simulink model "Docking"  (R2024b)
settings: Solver=VariableStepAuto  StartTime=0.0  StopTime=inf  RelTol=1e-3
values from neighbouring files (symbols this model uses):
  mu = 3.986e14    (= 398600000000000)    [DockSimParams.m]
undefined symbols (not defined in the file or in its folder): prox, sat
libraries: matrix_library x3
settings Model: Creator=Ameya  LastModifiedBy=Ameya
settings RTWCC: GPUComputeCapability=3.5

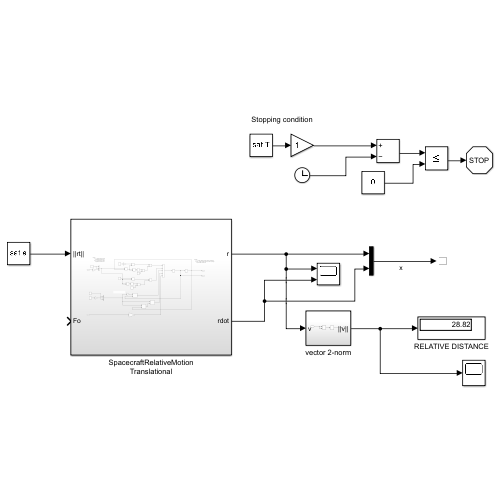
[thumbnail: Simulink's stored preview of the top-level diagram]
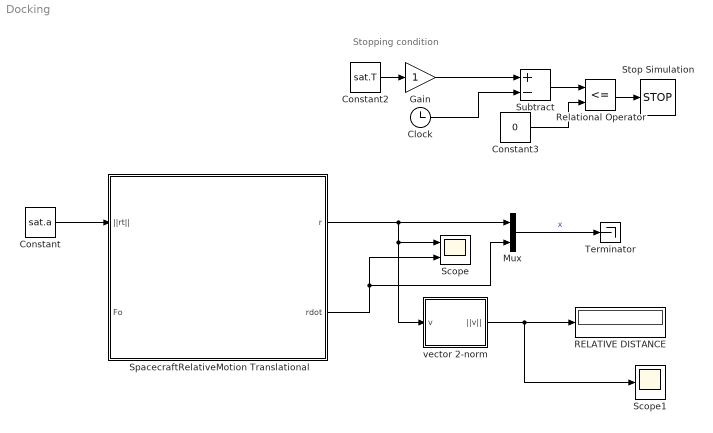
== system Docking ==
  note: Stopping condition
  Clock : Clock
  Constant : Constant  Value=sat.a
  Constant2 : Constant  Value=sat.T
  Constant3 : Constant  Value=0
  Gain : Gain
  Mux : Mux  Inputs=2
  RELATIVE DISTANCE : Display
  Relational Operator : RelationalOperator  Operator=<=  OutDataTypeStr=boolean  RndMeth=Simplest  InputSameDT=off
  Scope : Scope  NumInputPorts=2
  Scope1 : Scope
  SpacecraftRelativeMotion Translational : Subsystem
  Stop Simulation : Stop
  Subtract : Sum  Inputs=+-
  Terminator : Terminator
  vector 2-norm : Subsystem
  wires:
  SpacecraftRelativeMotion Translational/1(r) -> Mux/1, vector 2-norm/1(v), Scope/1
  SpacecraftRelativeMotion Translational/2(rdot) -> Mux/2, Scope/2
  Constant/1 -> SpacecraftRelativeMotion Translational/1(||rt||)
  Clock/1 -> Subtract/2
  Constant2/1 -> Gain/1
  Subtract/1 -> Relational Operator/1
  Constant3/1 -> Relational Operator/2
  Relational Operator/1 -> Stop Simulation/1
  vector 2-norm/1(||v||) -> RELATIVE DISTANCE/1, Scope1/1
  Gain/1 -> Subtract/1
  Mux/1 -> Terminator/1  "x"

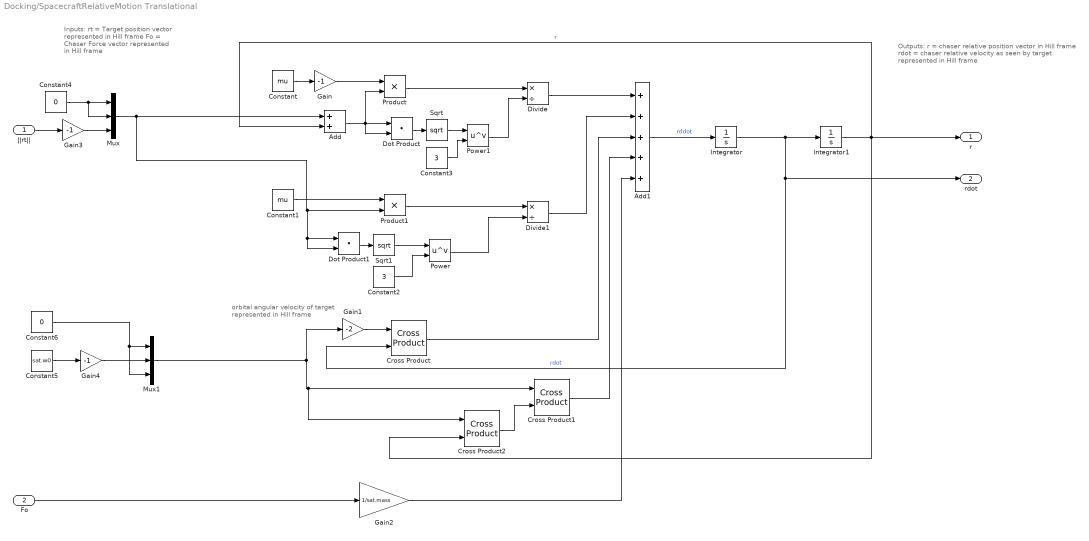
== system Docking/SpacecraftRelativeMotion Translational ==
  note: orbital angular velocity of target
      | represented in Hill frame
  note: Outputs:
      | r = chaser relative position vector in Hill frame
      | rdot = chaser relative velocity as seen by target
      | represented in Hill frame
  note: Inputs:
      | rt = Target position vector
      | represented in Hill frame
      | Fo = Chaser Force vector
      | represented in Hill frame
  ||rt|| : Inport
  Fo : Inport  Port=2
  Add : Sum
  Add1 : Sum  Inputs=+++++
  Constant : Constant  Value=mu
  Constant1 : Constant  Value=mu
  Constant2 : Constant  Value=3
  Constant3 : Constant  Value=3
  Constant4 : Constant  Value=0
  Constant5 : Constant  Value=sat.w0
  Constant6 : Constant  Value=0
  Cross Product : matrix_library/Cross Product
  Cross Product1 : matrix_library/Cross Product
  Cross Product2 : matrix_library/Cross Product
  Divide : Product  Inputs=*/
  Divide1 : Product  Inputs=*/
  Dot Product : DotProduct  OutDataTypeStr=Inherit: Inherit via internal rule
  Dot Product1 : DotProduct  OutDataTypeStr=Inherit: Inherit via internal rule
  Gain : Gain  Gain=-1
  Gain1 : Gain  Gain=-2
  Gain2 : Gain  Gain=1/sat.mass
  Gain3 : Gain  Gain=-1
  Gain4 : Gain  Gain=-1
  Integrator : Integrator  InitialCondition=prox.rdot
  Integrator1 : Integrator  InitialCondition=prox.r
  Mux : Mux  Inputs=3
  Mux1 : Mux  Inputs=3
  Power : Math  Operator=pow
  Power1 : Math  Operator=pow
  Product : Product
  Product1 : Product
  Sqrt : Sqrt
  Sqrt1 : Sqrt
  r : Outport
  rdot : Outport  Port=2
  wires:
  Mux1/1 -> Gain1/1, Cross Product2/1, Cross Product1/1
  Add/1 -> Dot Product/2, Product/2, Dot Product/1
  Power1/1 -> Divide/2
  Integrator/1 -> Integrator1/1, rdot/1, Cross Product/2  "rdot"
  Cross Product/1 -> Add1/3
  Dot Product1/1 -> Sqrt1/1
  Add1/1 -> Integrator/1  "rddot"
  Gain/1 -> Product/1
  Power/1 -> Divide1/2
  Product/1 -> Divide/1
  Cross Product2/1 -> Cross Product1/2
  Product1/1 -> Divide1/1
  Dot Product/1 -> Sqrt/1
  Gain1/1 -> Cross Product/1
  Constant/1 -> Gain/1
  Divide/1 -> Add1/1
  Integrator1/1 -> r/1, Add/2, Cross Product2/2  "r"
  Divide1/1 -> Add1/2
  Constant3/1 -> Power1/2
  Fo/1 -> Gain2/1
  Constant1/1 -> Product1/1
  Sqrt/1 -> Power1/1
  Sqrt1/1 -> Power/1
  Constant2/1 -> Power/2
  Gain2/1 -> Add1/5
  Cross Product1/1 -> Add1/4
  Mux/1 -> Add/1, Dot Product1/2, Dot Product1/1, Product1/2
  Gain3/1 -> Mux/3
  ||rt||/1 -> Gain3/1
  Constant4/1 -> Mux/1, Mux/2
  Constant6/1 -> Mux1/1, Mux1/3
  Gain4/1 -> Mux1/2
  Constant5/1 -> Gain4/1

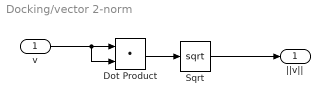
== system Docking/vector 2-norm ==
  v : Inport
  Dot Product : DotProduct  OutDataTypeStr=Inherit: Inherit via internal rule
  Sqrt : Sqrt
  ||v|| : Outport
  wires:
  Dot Product/1 -> Sqrt/1
  v/1 -> Dot Product/2, Dot Product/1
  Sqrt/1 -> ||v||/1
